simulink model "TaskD_MPC"  (R2022b)
settings: Solver=VariableStepAuto  StartTime=0.0  StopTime=10.0  RelTol=1e-3
undefined symbols (not defined in the file): A_11, A_12, A_21, A_22, absolute_encoder_counts_per_revolution, B_1, B_2, init, L_d, sample_time
libraries: simulink_extras x4, mpclib x1
settings Model: Creator=tumisangramotlhwa  LastModifiedBy=tumisangramotlhwa

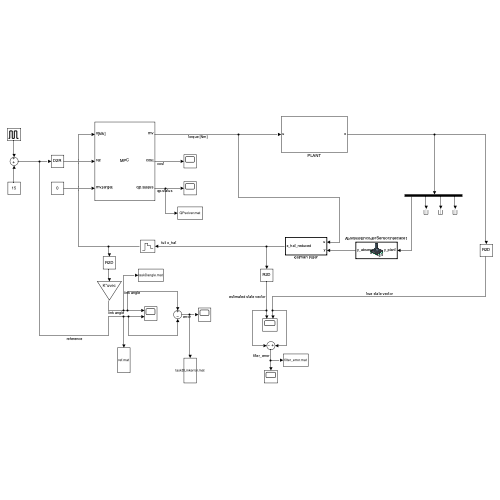
[thumbnail: Simulink's stored preview of the top-level diagram]
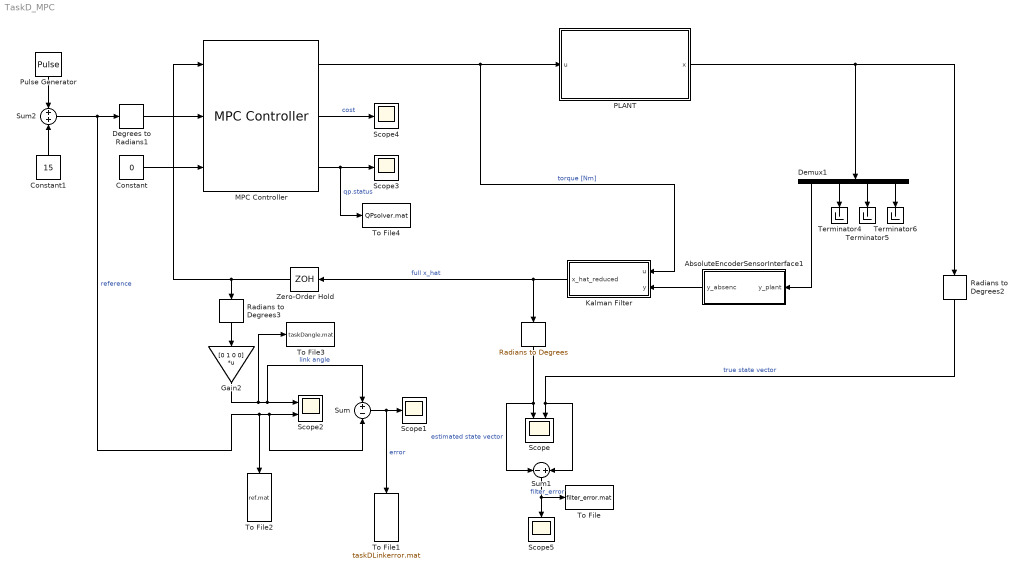
== system TaskD_MPC ==
  " " : simulink_extras/Transformations/Radians to Degrees
  AbsoluteEncoderSensorInterface1 : Subsystem  TreatAsAtomicUnit=on
      mask Display: image('$imagefile'); % Use "Edit Image" on toolstrip to change.
  Constant : Constant  Value=0
  Constant1 : Constant  Value=15
  Degrees to Radians1 : simulink_extras/Transformations/Degrees to Radians
  Demux1 : Demux
  Gain2 : Gain  Gain=[0 1 0 0]  Multiplication=Matrix(K*u) (u vector)
  Kalman Filter : Subsystem  TreatAsAtomicUnit=on
  MPC Controller : mpclib/MPC Controller  SCDEnableBlockLinearizationSpecification=on  mpcobj=mpc_obj  x0=mpc_initial_state  is_multiple=0  enable_value=0  return_u0=off  updateMPCinCallerWorkspace=on  md_inport=off  mv_inport=off  uref_inport=on  return_cost=on  return_mvseq=off  return_qpstatus=on  return_xseq=off  return_state=off  return_ovseq=off  state_inport=on  umin_inport=off  umax_inport=off  ymin_inport=off  ymax_inport=off  cc_inport=off  ywt_inport=off  uwt_inport=off  duwt_inport=off  rhoeps_inport=off  pm_inport=off  MaximumP=10  HorizonChoice=FixedHorizon  n_ts=0.02  n_p=10  n_mv=1  n_md=0  n_ud=0  n_mo=1  n_uo=0  BlockDataType=double  SampleTimeInherited=off  switch_inport=off
  PLANT : Subsystem
  Pulse Generator : DiscretePulseGenerator  PulseType=Time based  Amplitude=30  Period=4  PulseWidth=50
  Radians to Degrees2 : simulink_extras/Transformations/Radians to Degrees
  Radians to Degrees3 : simulink_extras/Transformations/Radians to Degrees
  Scope : Scope  NumInputPorts=2
  Scope{1,3..5} (4 alike) : Scope
  Scope2 : Scope  NumInputPorts=2
  Sum : Sum  Inputs=+|-
  Sum1 : Sum  Inputs=-|+
  Sum2 : Sum  Inputs=+|+
  Terminator4 : Terminator
  Terminator5 : Terminator
  Terminator6 : Terminator
  To File : ToFile  Filename=filter_error.mat  MatrixName=filter_error  SaveFormat=Timeseries
  To File1 : ToFile  Filename=taskDLinkerror.mat  MatrixName=taskDLinkerror  SaveFormat=Timeseries
  To File2 : ToFile  Filename=ref.mat  MatrixName=ref  SaveFormat=Timeseries
  To File3 : ToFile  Filename=taskDangle.mat  MatrixName=taskDangle  SaveFormat=Timeseries
  To File4 : ToFile  Filename=QPsolver.mat  MatrixName=QPsolver  SaveFormat=Timeseries
  Zero-Order Hold : ZeroOrderHold  SampleTime=sample_time
  wires:
  Degrees to Radians1/1 -> MPC Controller/2
  MPC Controller/1 -> PLANT/1(u), Kalman Filter/1(u)  "torque [Nm]"
  Constant/1 -> MPC Controller/3
  Sum2/1 -> Degrees to Radians1/1, To File2/1, Sum/2, Scope2/2  "reference"
  Constant1/1 -> Sum2/2
  Pulse Generator/1 -> Sum2/1
  Demux1/2 -> Terminator4/1
  PLANT/1(x) -> Demux1/1, Radians to Degrees2/1
  Demux1/4 -> Terminator6/1
  Demux1/3 -> Terminator5/1
  AbsoluteEncoderSensorInterface1/1(y_absenc) -> Kalman Filter/2(y)
  Demux1/1 -> AbsoluteEncoderSensorInterface1/1(y_plant)
  Kalman Filter/1(x_hat_reduced) -> Zero-Order Hold/1, " "/1  "full x_hat"
  Zero-Order Hold/1 -> MPC Controller/1, Radians to Degrees3/1
  " "/1 -> Sum1/1, Scope/1  "estimated state vector"
  Radians to Degrees2/1 -> Sum1/2, Scope/2  "true state vector"
  Gain2/1 -> To File3/1, Scope2/1, Sum/1  "link angle"
  Radians to Degrees3/1 -> Gain2/1
  Sum/1 -> To File1/1, Scope1/1  "error"
  MPC Controller/3 -> To File4/1, Scope3/1  "qp.status"
  MPC Controller/2 -> Scope4/1  "cost"
  Sum1/1 -> To File/1, Scope5/1  "filter_error"

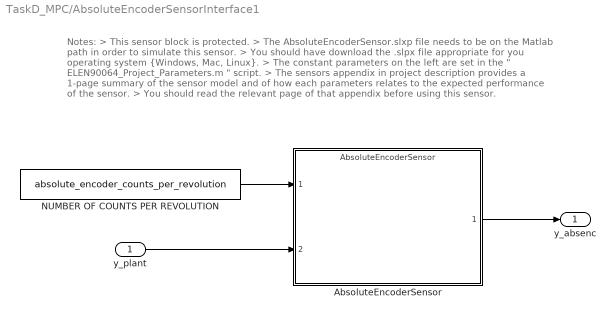
== system TaskD_MPC/AbsoluteEncoderSensorInterface1 ==
  note: Notes:
      | > This sensor block is protected.
      | > The AbsoluteEncoderSensor.slxp file needs to be on the Matlab path in order to simulate this sensor.
      | > You should have download the .slpx file appropriate for you operating system {Windows, Mac, Linux}.
      | > The constant parameters on the left are set in the " ELEN90064_Project_Parameters.m " script.
      | > The sensors appendix in project description provides a 1-page summary of the sensor model and of how each parameters relates to the expected performance of the sensor.
      | > You should read the relevant page of that appendix before using this sensor.
  y_plant : Inport
  AbsoluteEncoderSensor : ModelReference  ModelNameDialog=AbsoluteEncoderSensor.slxp  ModelReferenceVersion=1.16  CopyOfModelProtected=on
  NUMBER OF COUNTS PER REVOLUTION : Constant  Value=absolute_encoder_counts_per_revolution
  y_absenc : Outport
  wires:
  NUMBER OF COUNTS PER REVOLUTION/1 -> AbsoluteEncoderSensor/1
  y_plant/1 -> AbsoluteEncoderSensor/2
  AbsoluteEncoderSensor/1 -> y_absenc/1

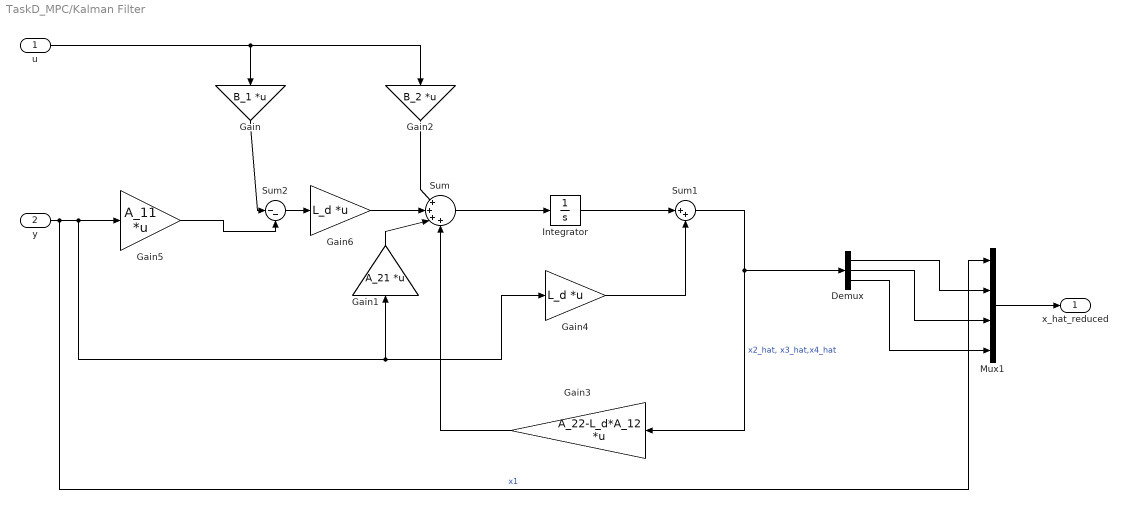
== system TaskD_MPC/Kalman Filter ==
  u : Inport
  y : Inport  Port=2
  Demux : Demux  Outputs=3
  Gain : Gain  Gain=B_1  Multiplication=Matrix(K*u) (u vector)
  Gain1 : Gain  Gain=A_21  Multiplication=Matrix(K*u) (u vector)
  Gain2 : Gain  Gain=B_2  Multiplication=Matrix(K*u) (u vector)
  Gain3 : Gain  Gain=A_22-L_d*A_12  Multiplication=Matrix(K*u) (u vector)
  Gain4 : Gain  Gain=L_d  Multiplication=Matrix(K*u) (u vector)
  Gain5 : Gain  Gain=A_11  Multiplication=Matrix(K*u) (u vector)
  Gain6 : Gain  Gain=L_d  Multiplication=Matrix(K*u) (u vector)
  Integrator : Integrator
  Mux1 : Mux
  Sum : Sum  Inputs=|++++
  Sum1 : Sum  Inputs=|++
  Sum2 : Sum  Inputs=|--
  x_hat_reduced : Outport
  wires:
  u/1 -> Gain2/1, Gain/1
  y/1 -> Mux1/1, Gain5/1, Gain4/1, Gain1/1  "x1"
  Sum/1 -> Integrator/1
  Gain6/1 -> Sum/2
  Gain1/1 -> Sum/3
  Gain/1 -> Sum2/1
  Gain5/1 -> Sum2/2
  Gain2/1 -> Sum/1
  Integrator/1 -> Sum1/1
  Gain4/1 -> Sum1/2
  Gain3/1 -> Sum/4
  Sum1/1 -> Demux/1, Gain3/1  "x2_hat, x3_hat,x4_hat"
  Sum2/1 -> Gain6/1
  Mux1/1 -> x_hat_reduced/1
  Demux/1 -> Mux1/2
  Demux/2 -> Mux1/3
  Demux/3 -> Mux1/4

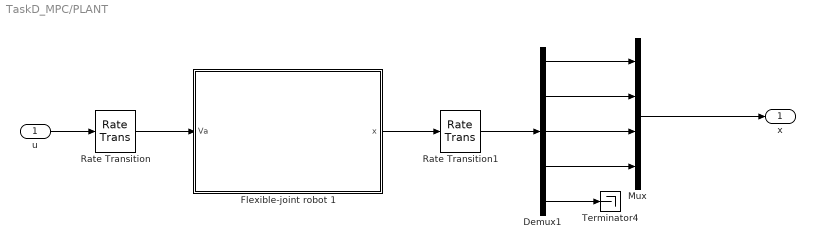
== system TaskD_MPC/PLANT ==
  u : Inport
  Demux1 : Demux  Outputs=5
  Flexible-joint robot 1 : Subsystem
      mask Display: image('$imagefile'); % Use "Edit Image" on toolstrip to change.
  Mux : Mux
  Rate Transition : RateTransition  OutPortSampleTime=0.02
  Rate Transition1 : RateTransition  OutPortSampleTime=0.02
  Terminator4 : Terminator
  x : Outport
  wires:
  Demux1/4 -> Mux/4
  Demux1/3 -> Mux/3
  Demux1/2 -> Mux/2
  Demux1/1 -> Mux/1
  Demux1/5 -> Terminator4/1
  u/1 -> Rate Transition/1
  Mux/1 -> x/1
  Flexible-joint robot 1/1(x) -> Rate Transition1/1
  Rate Transition1/1 -> Demux1/1
  Rate Transition/1 -> Flexible-joint robot 1/1(Va)

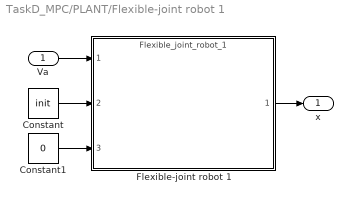
== system TaskD_MPC/PLANT/Flexible-joint robot 1 ==
  Va : Inport
  Constant : Constant  Value=init
  Constant1 : Constant  Value=0
  Flexible-joint robot 1 : ModelReference  ModelNameDialog=Flexible_joint_robot_1  ModelReferenceVersion=1.63  CopyOfModelProtected=on
  x : Outport
  wires:
  Constant/1 -> Flexible-joint robot 1/2
  Constant1/1 -> Flexible-joint robot 1/3
  Flexible-joint robot 1/1 -> x/1
  Va/1 -> Flexible-joint robot 1/1
